simulink model "U21EE081"  (R2014a)
settings: Solver=ode23t  StartTime=0.0  StopTime=0.02  RelTol=1e-3
libraries: powerlib x13
settings Model: Creator=dell  LastModifiedBy=dell

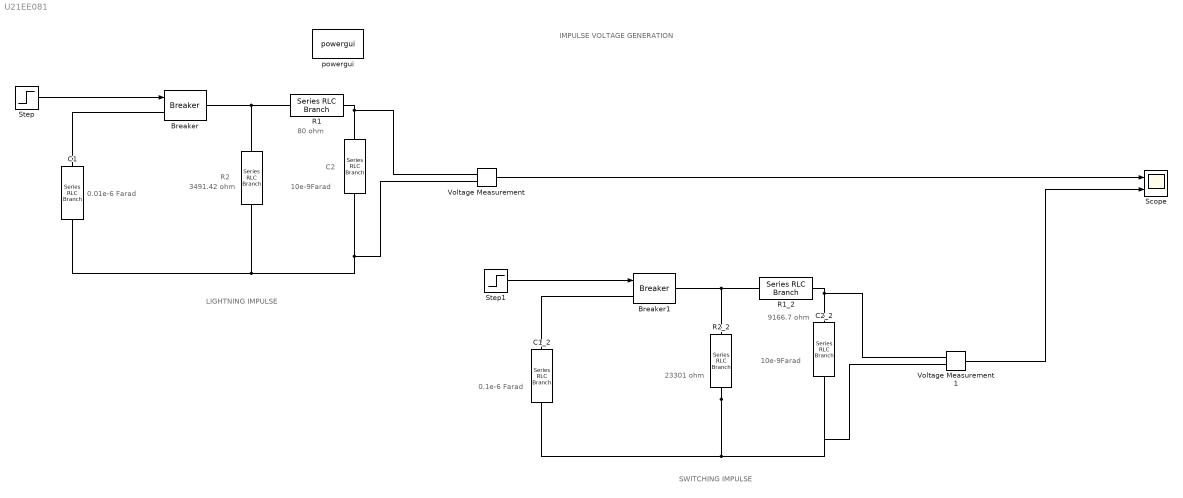
== system U21EE081 ==
  note: 10e-9Farad
  note: 9166.7 ohm
  note: 23301 ohm
  note: 0.1e-6 Farad
  note: C2
  note: R2
  note: 10e-9Farad
  note: 3491.42 ohm
  note: 80 ohm
  note: 0.01e-6 Farad
  note: SWITCHING IMPULSE
  note: LIGHTNING IMPULSE
  note: IMPULSE VOLTAGE GENERATION
  " " : powerlib/Elements/Series RLC Branch  LConnTagsString=__new0  RConnTagsString=__new0  BranchType=R  Resistance=3491.42  Inductance=1e-3  SetiL0=off  InitialCurrent=0  Capacitance=1e-6  Setx0=off  InitialVoltage=0  Measurements=None
  " " : powerlib/Elements/Series RLC Branch  LConnTagsString=__new0  RConnTagsString=__new0  BranchType=C  Resistance=1  Inductance=1e-3  SetiL0=off  InitialCurrent=0  Capacitance=10e-9  Setx0=off  InitialVoltage=0  Measurements=Branch voltage
  Breaker : powerlib/Elements/Breaker  InitialState=0  SwitchingTimes="[1/60  5/60]"  External=on  BreakerResistance=0.01  SnubberResistance=1e6  SnubberCapacitance=inf  Measurements=None  MoreParameters=on  NoBreakLoop=off
  Breaker1 : powerlib/Elements/Breaker  InitialState=0  SwitchingTimes="[1/60  5/60]"  External=on  BreakerResistance=0.01  SnubberResistance=1e6  SnubberCapacitance=inf  Measurements=None  MoreParameters=on  NoBreakLoop=off
  C1 : powerlib/Elements/Series RLC Branch  LConnTagsString=__new0  RConnTagsString=__new0  BranchType=C  Resistance=1  Inductance=1e-3  SetiL0=off  InitialCurrent=0  Capacitance=0.01e-6  Setx0=on  InitialVoltage=100000  Measurements=None
  C1_2 : powerlib/Elements/Series RLC Branch  LConnTagsString=__new0  RConnTagsString=__new0  BranchType=C  Resistance=1  Inductance=1e-3  SetiL0=off  InitialCurrent=0  Capacitance=0.1e-6  Setx0=on  InitialVoltage=100e3  Measurements=None
  C2_2 : powerlib/Elements/Series RLC Branch  LConnTagsString=__new0  RConnTagsString=__new0  BranchType=C  Resistance=1  Inductance=1e-3  SetiL0=off  InitialCurrent=0  Capacitance=10e-9  Setx0=off  InitialVoltage=0  Measurements=Branch voltage
  R1 : powerlib/Elements/Series RLC Branch  LConnTagsString=__new0  RConnTagsString=__new0  BranchType=R  Resistance=80  Inductance=1e-3  SetiL0=off  InitialCurrent=0  Capacitance=1e-6  Setx0=off  InitialVoltage=0  Measurements=None
  R1_2 : powerlib/Elements/Series RLC Branch  LConnTagsString=__new0  RConnTagsString=__new0  BranchType=R  Resistance=9166.7  Inductance=1e-3  SetiL0=off  InitialCurrent=0  Capacitance=1e-6  Setx0=off  InitialVoltage=0  Measurements=None
  R2_2 : powerlib/Elements/Series RLC Branch  LConnTagsString=__new0  RConnTagsString=__new0  BranchType=R  Resistance=23301  Inductance=1e-3  SetiL0=off  InitialCurrent=0  Capacitance=1e-6  Setx0=off  InitialVoltage=0  Measurements=None
  Scope : Scope  NumInputPorts=2
      settings: YMin=-5~-5  YMax=5~5
  Step : Step  Time=0.001  SampleTime=0
  Step1 : Step  Time=0.001  SampleTime=0
  Voltage Measurement : powerlib/Measurements/Voltage Measurement  PhasorSimulation=off  OutputType=Complex  PSBequivalent=0
  Voltage Measurement1 : powerlib/Measurements/Voltage Measurement  PhasorSimulation=off  OutputType=Complex  PSBequivalent=0
  powergui : powerlib/powergui  Priority=1  SimulationMode=Continuous  SolverType=Tustin  SampleTime=50e-6  frequency=60  SPID=off  DisableSnubberDevices=off  DisableRonSwitches=off  DisableVfSwitches=off  SwTol=0  Interpol=off  DisplayEquations=off  Ts=0  methode=off  frequencyindice=0  Pbase=100e6  ErrMax=1e-4  Iterations=50  UnitsV=kV  UnitsW=MW  FunctionMessages=off  echomessages=off  HookPort=off  EnableUseOfTLC=off  x0status=blocks  RestoreLinks=warning  ResistiveCurrentMeasurement=off  Frange=[0:2:500]  Ylog=off  Xlog=on  ShowGrid=off  save=off  variable=ZData  structure=0  ZoomFFT=off  StartTime=0.0  cycles=1  DisplayStyle=1  fundamental=60  FreqAxis=off  MaxFrequency=1000  frequencyindicesteady=1  RmsSteady=1  display=off
  wires:
  Voltage Measurement/1 -> Scope/1
  Step/1 -> Breaker/1
  Step1/1 -> Breaker1/1
  Voltage Measurement1/1 -> Scope/2
  connections:
  R1/LConn1 -- Voltage Measurement/LConn1 -- " "/LConn1
  Breaker/RConn1 -- " "/LConn1 -- R1/RConn1
  " "/RConn1 -- Voltage Measurement/LConn2 -- C1/RConn1
  C1/LConn1 -- Breaker/LConn1
  R1_2/LConn1 -- Voltage Measurement1/LConn1 -- C2_2/LConn1
  Breaker1/RConn1 -- R2_2/LConn1 -- R1_2/RConn1
  R2_2/RConn1 -- C1_2/RConn1 -- C2_2/RConn1 -- Voltage Measurement1/LConn2
  C1_2/LConn1 -- Breaker1/LConn1
